simulink model "Traction_control_system_block"  (R2024b)
settings: Solver=VariableStepAuto  StartTime=0.0  StopTime=10.0  RelTol=1e-3
libraries: spspowerguiLib x1
settings Model: Creator=abdula  LastModifiedBy=abdula

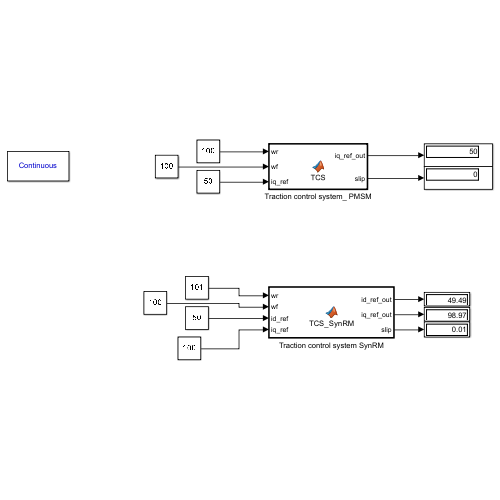
[thumbnail: Simulink's stored preview of the top-level diagram]
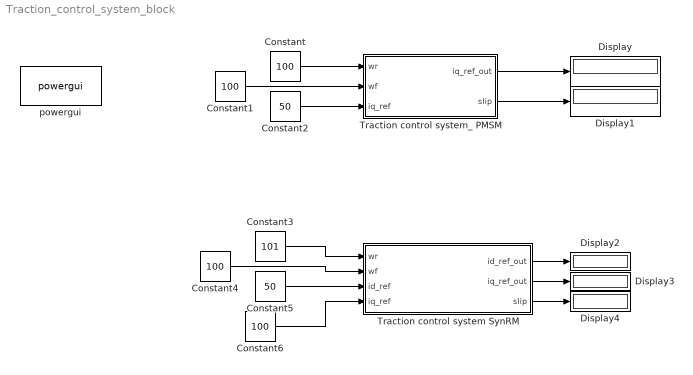
== system Traction_control_system_block ==
  Constant{,1,4,6} (4 alike) : Constant  Value=100
  Constant2 : Constant  Value=50
  Constant3 : Constant  Value=101
  Constant5 : Constant  Value=50
  Display{,1..4} (5 alike) : Display
  Traction control system SynRM : MATLAB Function  TreatAsAtomicUnit=on
  Traction control system_ PMSM : MATLAB Function  TreatAsAtomicUnit=on
  powergui : spspowerguiLib/powergui  Priority=1  SimulationMode=Continuous  SampleTime=50e-6  frequency=60  Iterations=50  frequencyindice=60  Pbase=100e6  ErrMax=1e-4  UnitsV=kV  UnitsW=MW  buscounter=0  FunctionMessages=off  echomessages=off  EnableUseOfTLC=off  CurrentSourceSwitches=off  DisableSnubberDevices=off  DisableRonSwitches=off  DisableVfSwitches=off  DisplayEquations=off  AutomaticDiscreteSolvers=off  SolverType=Tustin/Backward Euler (TBE)  Interpol=off  ExternalGateDelay=off  methode=off  Ts=100  x0status=blocks  SPID=on  SwTol=0  HookPort=off  NonlinearTolerance=1e-4  nMaxIteration=100  ContinueOnMaxIteration=off  RestoreLinks=warning  ResistiveCurrentMeasurement=off  Frange=[0:2:500]  Ylog=off  Xlog=on  ShowGrid=off  save=off  variable=ZData  structure=0  ZoomFFT=off  StartTime=0.0  cycles=1  DisplayStyle=1  fundamental=60  FreqAxis=off  MaxFrequency=1000  frequencyindicesteady=1  RmsSteady=1  display=off
  wires:
  Constant/1 -> Traction control system_ PMSM/1(wr)
  Constant1/1 -> Traction control system_ PMSM/2(wf)
  Constant2/1 -> Traction control system_ PMSM/3(iq_ref)
  Traction control system_ PMSM/1(iq_ref_out) -> Display/1
  Traction control system_ PMSM/2(slip) -> Display1/1
  Constant5/1 -> Traction control system SynRM/3(id_ref)
  Constant4/1 -> Traction control system SynRM/2(wf)
  Constant3/1 -> Traction control system SynRM/1(wr)
  Constant6/1 -> Traction control system SynRM/4(iq_ref)
  Traction control system SynRM/1(id_ref_out) -> Display2/1
  Traction control system SynRM/2(iq_ref_out) -> Display3/1
  Traction control system SynRM/3(slip) -> Display4/1

== matlab function Traction_control_system_block/Traction control system SynRM ==
  data: id_ref_out output; wr input; iq_ref_out output; wf input; id_ref input; iq_ref input; slip output
function [id_ref_out, iq_ref_out, slip] = TCS_SynRM( ...
                                wr, wf, id_ref, iq_ref)

% =========================================================
% SynRM Traction Control (Current Scaling Method)
% No MTPA
% No torque model
% Reduce BOTH id and iq proportionally
% Codegen compatible
% =========================================================

%% ===== PARAMETERS =====
Kp = 2;
Ki = 200;

slip_ref  = 0.005;     % 0.5 %
deadband  = 0.0005;
min_speed = 1;         % rad/s
Ts = 5e-6;

max_scale_reduction = 1;   % full cut allowed id,id=0

%% ===== PERSISTENT =====
persistent integ
if isempty(integ)
    integ = 0;
end

%% ===== SLIP =====
eps_speed = 1e-3;
den = max(abs(wf), eps_speed);

slip = (wr - wf) / den;

%% ===== DISABLE AT LOW SPEED =====
if abs(wf) < min_speed
    id_ref_out = id_ref;
    iq_ref_out = iq_ref;
    integ = 0;
    return
end

%% ===== ERROR =====
if abs(slip) < deadband
    error = 0;
else
    error = slip - slip_ref;
end

%% ===== PI CONTROLLER =====
integ = integ + Ki * error * Ts;

delta = Kp * error + integ;

% only reduce torque (no boost)
delta = max(delta, 0);

% clamp
delta = min(delta, max_scale_reduction);

%% ===== SCALE FACTOR =====
alpha = 1 - delta;

alpha = min(max(alpha,0),1);

%% ===== CURRENT REDUCTION =====
id_ref_out = alpha * id_ref;
iq_ref_out = alpha * iq_ref;

end

== matlab function Traction_control_system_block/Traction control system_ PMSM ==
  data: wr input; iq_ref_out output; wf input; iq_ref input; slip output
function [iq_ref_out, slip] = TCS(wr, wf, iq_ref)
% =========================================================
% Traction Control System for Two-Wheeler EV
% Slip-based torque reduction
% Codegen compatible
% =========================================================

%% ===== USER PARAMETERS =====
Kp = 30;                 % proportional gain
Ki = 300;                % integral gain
slip_ref = 0.005;         % 0.5% desired slip
deadband = 0.0005;         % 0.05% ignore small slip
iq_max_reduction = 150;  % max current reduction (A)
min_speed = 1;           % disable TCS below this (rad/s)
Ts =5e-6;                % sample time (sec)

%% ===== PERSISTENT STATES =====
persistent integ
if isempty(integ)
    integ = 0;
end

%% ===== SLIP CALCULATION =====
eps_speed = 1e-3;
den = max(abs(wf), eps_speed);

slip = (wr - wf) / den;

%% ===== DISABLE AT LOW SPEED =====
if abs(wf) < min_speed
    iq_ref_out = iq_ref;
    integ = 0;
    return
end

%% ===== DEAD BAND =====
if abs(slip) < deadband
    error = 0;
else
    error = slip - slip_ref;
end

%% ===== PI CONTROLLER =====
integ = integ + Ki * error * Ts;

% anti-windup clamp
integ = min(max(integ, -iq_max_reduction), iq_max_reduction);

delta_iq = Kp * error + integ;

% only reduce torque (no positive addition)
delta_iq = max(delta_iq, 0);

% clamp reduction
delta_iq = min(delta_iq, iq_max_reduction);

%% ===== OUTPUT =====
iq_ref_out = iq_ref - delta_iq;

end
